simulink model "test_ab_to_ae"  (Simulink 7.6)
settings: Solver=ode45  StartTime=0.0  StopTime=500  RelTol=1e-3
libraries: simulink x18
settings Model: Creator=jporter  LastModifiedBy=jporter

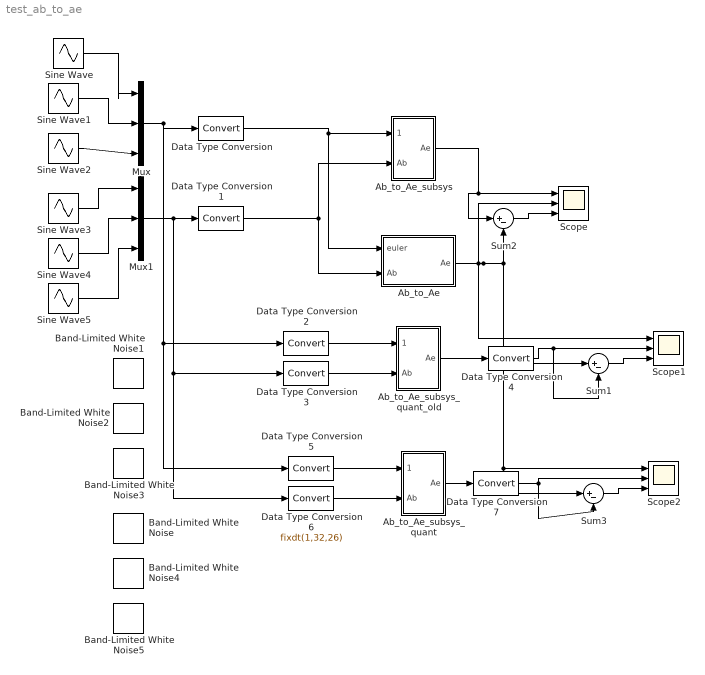
== system test_ab_to_ae ==
  Ab_to_Ae : Stateflow chart  TreatAsAtomicUnit=on
  Ab_to_Ae_subsys : Subsystem
  Ab_to_Ae_subsys_quant : Subsystem
  Ab_to_Ae_subsys_quant_old : Subsystem
  Band-Limited White Noise : simulink/Sources/Band-Limited White Noise  SystemSampleTime=-1  Cov=0.5  Ts=0.01  seed=[23341]
  Band-Limited White Noise{1..3,5} (4 alike) : simulink/Sources/Band-Limited White Noise  SystemSampleTime=-1  Cov=0  Ts=0.01  seed=[23341]
  Band-Limited White Noise4 : simulink/Sources/Band-Limited White Noise  SystemSampleTime=-1  Cov=0.5  Ts=0.01  seed=[23341]
  Data Type Conversion{,1..5,7} (7 alike) : DataTypeConversion
  Data Type Conversion6 : DataTypeConversion  OutDataTypeStr=fixdt(1,32,26)
  Mux : Mux  Inputs=3
  Mux1 : Mux  Inputs=3
  Scope : Scope  NumInputPorts=3
      settings: YMin=-5~-5~-5  YMax=5~5~5
  Scope1 : Scope  NumInputPorts=3
      settings: YMin=-1.5~-1.25~-2  YMax=1.5~0.75~1.5
  Scope2 : Scope  NumInputPorts=3
      settings: YMin=-1.25~-1.25~-7.5e-005  YMax=1.25~1.25~7.5e-005  SaveName=ScopeData2
  Sine Wave : Sin  SampleTime=0
  Sine Wave1 : Sin  Phase=1  SampleTime=0
  Sine Wave2 : Sin  Phase=2  SampleTime=0
  Sine Wave3 : Sin  Phase=3  SampleTime=0
  Sine Wave4 : Sin  Phase=4  SampleTime=0
  Sine Wave5 : Sin  Phase=5  SampleTime=0
  Sum1 : Sum  Inputs=|+-
  Sum2 : Sum  Inputs=|+-
  Sum3 : Sum  Inputs=|+-
  wires:
  Ab_to_Ae_subsys/1(Ae) -> Scope/1, Sum2/1
  Ab_to_Ae/1(Ae) -> Scope/2, Scope1/1, Sum2/2, Sum1/1, Scope2/1, Sum3/1
  Mux/1 -> Data Type Conversion/1, Data Type Conversion2/1, Data Type Conversion5/1
  Mux1/1 -> Data Type Conversion1/1, Data Type Conversion3/1, Data Type Conversion6/1
  Data Type Conversion/1 -> Ab_to_Ae_subsys/1(euler), Ab_to_Ae/1(euler)
  Data Type Conversion1/1 -> Ab_to_Ae/2(Ab), Ab_to_Ae_subsys/2(Ab)
  Sum2/1 -> Scope/3
  Sine Wave/1 -> Mux/1
  Sine Wave1/1 -> Mux/2
  Sine Wave2/1 -> Mux/3
  Sine Wave3/1 -> Mux1/1
  Sine Wave4/1 -> Mux1/2
  Sine Wave5/1 -> Mux1/3
  Data Type Conversion2/1 -> Ab_to_Ae_subsys_quant_old/1(euler)
  Data Type Conversion3/1 -> Ab_to_Ae_subsys_quant_old/2(Ab)
  Ab_to_Ae_subsys_quant_old/1(Ae) -> Data Type Conversion4/1
  Data Type Conversion4/1 -> Scope1/2, Sum1/2
  Sum1/1 -> Scope1/3
  Ab_to_Ae_subsys_quant/1(Ae) -> Data Type Conversion7/1
  Sum3/1 -> Scope2/3
  Data Type Conversion5/1 -> Ab_to_Ae_subsys_quant/1(euler1)
  Data Type Conversion6/1 -> Ab_to_Ae_subsys_quant/2(Ab)
  Data Type Conversion7/1 -> Scope2/2, Sum3/2

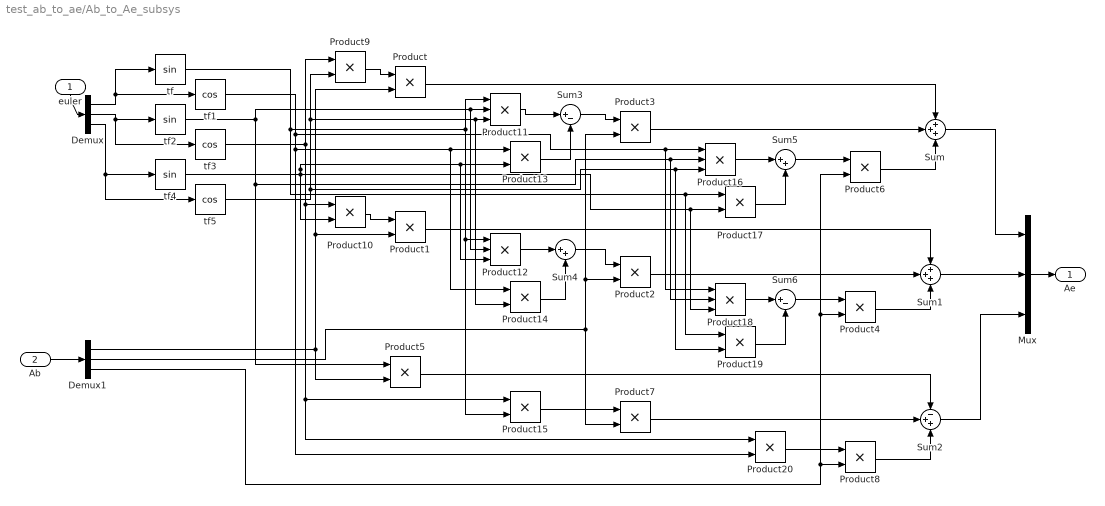
== system test_ab_to_ae/Ab_to_Ae_subsys ==
  euler : Inport
  Ab : Inport  Port=2
  Demux : Demux  Outputs=3
  Demux1 : Demux  Outputs=3
  Mux : Mux  Inputs=3
  Product{,1..10,13..15,17,19..20} (17 alike) : Product  RndMeth=Zero
  Product{11..12,16,18} (4 alike) : Product  Inputs=3  RndMeth=Zero
  Sum : Sum  Inputs=+++
  Sum1 : Sum  Inputs=+++
  Sum2 : Sum  Inputs=-++
  Sum3 : Sum  Inputs=|+-
  Sum4 : Sum  Inputs=|++
  Sum5 : Sum  Inputs=|++
  Sum6 : Sum  Inputs=|+-
  tf : Trigonometry
  tf1 : Trigonometry  Operator=cos
  tf2 : Trigonometry
  tf3 : Trigonometry  Operator=cos
  tf4 : Trigonometry
  tf5 : Trigonometry  Operator=cos
  Ae : Outport
  wires:
  Demux/1 -> tf/1, tf1/1
  Demux/2 -> tf2/1, tf3/1
  Demux/3 -> tf4/1, tf5/1
  Product/1 -> Sum/1
  Product3/1 -> Sum/2
  Product6/1 -> Sum/3
  Product1/1 -> Sum1/1
  Product2/1 -> Sum1/2
  Product4/1 -> Sum1/3
  Product5/1 -> Sum2/1
  Product7/1 -> Sum2/2
  Product8/1 -> Sum2/3
  tf3/1 -> Product9/1, Product10/1, Product15/1, Product20/1
  tf5/1 -> Product9/2, Product11/3, Product14/2, Product16/3, Product19/2
  Product9/1 -> Product/1
  Demux1/1 -> Product/2, Product1/2, Product5/2
  tf4/1 -> Product10/2, Product13/2, Product12/3, Product17/2, Product18/3
  Product10/1 -> Product1/1
  tf2/1 -> Product11/2, Product12/2, Product5/1, Product16/2, Product18/2
  Product11/1 -> Sum3/1
  tf/1 -> Product11/1, Product12/1, Product15/2, Product17/1, Product19/1
  tf1/1 -> Product16/1, Product18/1, Product13/1, Product14/1, Product20/2
  Product13/1 -> Sum3/2
  Sum3/1 -> Product3/1
  Demux1/2 -> Product3/2, Product2/2, Product7/2
  Product12/1 -> Sum4/1
  Product14/1 -> Sum4/2
  Sum4/1 -> Product2/1
  Product15/1 -> Product7/1
  Product16/1 -> Sum5/1
  Product17/1 -> Sum5/2
  Product18/1 -> Sum6/1
  Product19/1 -> Sum6/2
  Sum5/1 -> Product6/1
  Sum6/1 -> Product4/1
  Product20/1 -> Product8/1
  Demux1/3 -> Product8/2, Product4/2, Product6/2
  Sum/1 -> Mux/1
  Sum1/1 -> Mux/2
  Sum2/1 -> Mux/3
  euler/1 -> Demux/1
  Ab/1 -> Demux1/1
  Mux/1 -> Ae/1

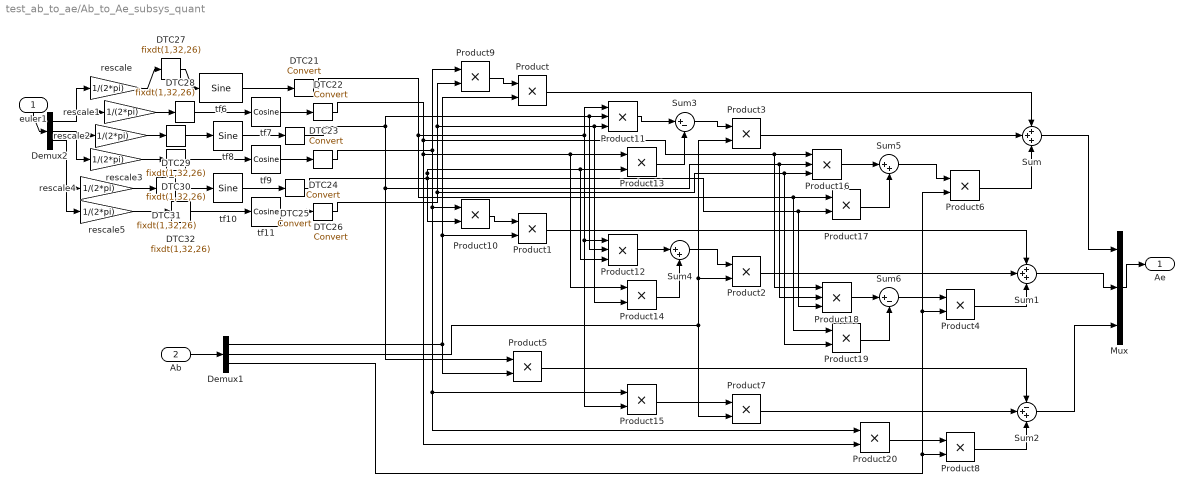
== system test_ab_to_ae/Ab_to_Ae_subsys_quant ==
  euler1 : Inport
  Ab : Inport  Port=2
  DTC{21..26} (6 alike) : DataTypeConversion
  DTC{27..32} (6 alike) : DataTypeConversion  OutDataTypeStr=fixdt(1,32,26)
  Demux1 : Demux  Outputs=3
  Demux2 : Demux  Outputs=3
  Mux : Mux  Inputs=3
  Product{,1..10,13..15,17,19..20} (17 alike) : Product  OutDataTypeStr=Inherit: Inherit via back propagation  RndMeth=Zero
  Product{11..12,16,18} (4 alike) : Product  Inputs=3  OutDataTypeStr=Inherit: Inherit via back propagation  RndMeth=Zero
  Sum : Sum  Inputs=+++  OutDataTypeStr=Inherit: Inherit via back propagation
  Sum1 : Sum  Inputs=+++  OutDataTypeStr=Inherit: Inherit via back propagation
  Sum2 : Sum  Inputs=-++  OutDataTypeStr=Inherit: Inherit via back propagation
  Sum3 : Sum  Inputs=|+-  OutDataTypeStr=Inherit: Inherit via back propagation
  Sum4 : Sum  Inputs=|++  OutDataTypeStr=Inherit: Inherit via back propagation
  Sum5 : Sum  Inputs=|++  OutDataTypeStr=Inherit: Inherit via back propagation
  Sum6 : Sum  Inputs=|+-  OutDataTypeStr=Inherit: Inherit via back propagation
  rescale{,1..5} (6 alike) : Gain  Gain=1/(2*pi)  ParamMin=1/(2*pi)  ParamMax=1/(2*pi)  OutDataTypeStr=fixdt(1,64,58)
  tf10 : simulink/Lookup Tables/Sine  SystemSampleTime=-1  Formula=sin(2*pi*u)  NumDataPoints=(2^7)+1  OutputWordLength=32
  tf11 : simulink/Lookup Tables/Cosine  SystemSampleTime=-1  Formula=cos(2*pi*u)  NumDataPoints=(2^7)+1  OutputWordLength=32
  tf6 : simulink/Lookup Tables/Sine  SystemSampleTime=-1  Formula=sin(2*pi*u)  NumDataPoints=(2^7)+1  OutputWordLength=32
  tf7 : simulink/Lookup Tables/Cosine  SystemSampleTime=-1  Formula=cos(2*pi*u)  NumDataPoints=(2^7)+1  OutputWordLength=32
  tf8 : simulink/Lookup Tables/Sine  SystemSampleTime=-1  Formula=sin(2*pi*u)  NumDataPoints=(2^7)+1  OutputWordLength=32
  tf9 : simulink/Lookup Tables/Cosine  SystemSampleTime=-1  Formula=cos(2*pi*u)  NumDataPoints=(2^7)+1  OutputWordLength=32
  Ae : Outport
  wires:
  Product/1 -> Sum/1
  Product3/1 -> Sum/2
  Product6/1 -> Sum/3
  Product1/1 -> Sum1/1
  Product2/1 -> Sum1/2
  Product4/1 -> Sum1/3
  Product5/1 -> Sum2/1
  Product7/1 -> Sum2/2
  Product8/1 -> Sum2/3
  DTC24/1 -> Product9/1, Product10/1, Product15/1, Product20/1
  DTC26/1 -> Product9/2, Product11/3, Product14/2, Product16/3, Product19/2
  Product9/1 -> Product/1
  Demux1/1 -> Product/2, Product1/2, Product5/2
  DTC25/1 -> Product10/2, Product13/2, Product12/3, Product17/2, Product18/3
  Product10/1 -> Product1/1
  DTC23/1 -> Product11/2, Product12/2, Product5/1, Product16/2, Product18/2
  Product11/1 -> Sum3/1
  DTC21/1 -> Product11/1, Product15/2, Product12/1, Product17/1, Product19/1
  DTC22/1 -> Product16/1, Product18/1, Product13/1, Product14/1, Product20/2
  Product13/1 -> Sum3/2
  Sum3/1 -> Product3/1
  Demux1/2 -> Product3/2, Product2/2, Product7/2
  Product12/1 -> Sum4/1
  Product14/1 -> Sum4/2
  Sum4/1 -> Product2/1
  Product15/1 -> Product7/1
  Product16/1 -> Sum5/1
  Product17/1 -> Sum5/2
  Product18/1 -> Sum6/1
  Product19/1 -> Sum6/2
  Sum5/1 -> Product6/1
  Sum6/1 -> Product4/1
  Product20/1 -> Product8/1
  Demux1/3 -> Product8/2, Product4/2, Product6/2
  Sum/1 -> Mux/1
  Sum1/1 -> Mux/2
  Sum2/1 -> Mux/3
  Ab/1 -> Demux1/1
  Mux/1 -> Ae/1
  Demux2/1 -> rescale/1, rescale1/1
  Demux2/2 -> rescale2/1, rescale3/1
  Demux2/3 -> rescale4/1, rescale5/1
  tf9/1 -> DTC24/1
  tf11/1 -> DTC26/1
  tf10/1 -> DTC25/1
  tf8/1 -> DTC23/1
  tf6/1 -> DTC21/1
  tf7/1 -> DTC22/1
  euler1/1 -> Demux2/1
  rescale/1 -> DTC27/1
  DTC27/1 -> tf6/1
  rescale1/1 -> DTC28/1
  DTC28/1 -> tf7/1
  rescale2/1 -> DTC29/1
  DTC29/1 -> tf8/1
  rescale3/1 -> DTC30/1
  DTC30/1 -> tf9/1
  rescale4/1 -> DTC31/1
  DTC31/1 -> tf10/1
  rescale5/1 -> DTC32/1
  DTC32/1 -> tf11/1

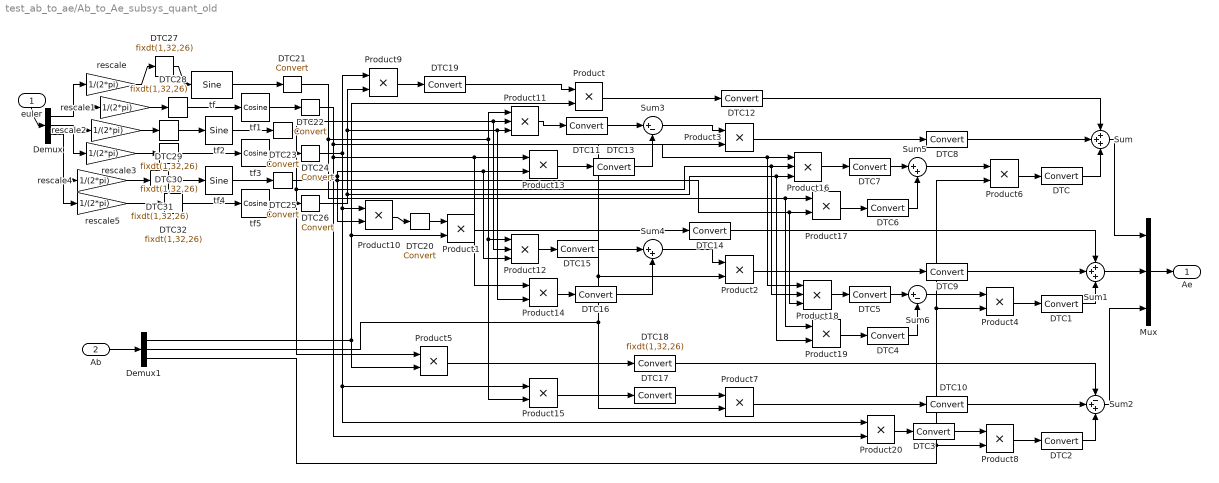
== system test_ab_to_ae/Ab_to_Ae_subsys_quant_old ==
  euler : Inport
  Ab : Inport  Port=2
  DTC{,1..17,19..26} (26 alike) : DataTypeConversion
  DTC{18,27..32} (7 alike) : DataTypeConversion  OutDataTypeStr=fixdt(1,32,26)
  Demux : Demux  Outputs=3
  Demux1 : Demux  Outputs=3
  Mux : Mux  Inputs=3
  Product : Product  OutDataTypeStr=fixdt(1,32,33)  RndMeth=Zero
  Product1 : Product  OutDataTypeStr=fixdt(1,32,34)  RndMeth=Zero
  Product{5,9..10,15} (4 alike) : Product  OutDataTypeStr=fixdt(1,64,52)  RndMeth=Zero
  Product11 : Product  Inputs=3  OutDataTypeStr=fixdt(1,64,52)  RndMeth=Zero
  Product12 : Product  Inputs=3  OutDataTypeStr=fixdt(1,32,41)  RndMeth=Zero
  Product13 : Product  OutDataTypeStr=fixdt(1,32,31)  RndMeth=Zero
  Product14 : Product  OutDataTypeStr=fixdt(1,32,30)  RndMeth=Zero
  Product16 : Product  Inputs=3  OutDataTypeStr=fixdt(1,32,35)  RndMeth=Zero
  Product17 : Product  OutDataTypeStr=fixdt(1,32,36)  RndMeth=Zero
  Product18 : Product  Inputs=3  OutDataTypeStr=fixdt(1,32,35)  RndMeth=Zero
  Product19 : Product  OutDataTypeStr=fixdt(1,32,35)  RndMeth=Zero
  Product2 : Product  OutDataTypeStr=fixdt(1,32,33)  RndMeth=Zero
  Product20 : Product  OutDataTypeStr=fixdt(1,32,30)  RndMeth=Zero
  Product3 : Product  OutDataTypeStr=fixdt(1,32,34)  RndMeth=Zero
  Product4 : Product  OutDataTypeStr=fixdt(1,32,39)  RndMeth=Zero
  Product6 : Product  OutDataTypeStr=fixdt(1,32,39)  RndMeth=Zero
  Product7 : Product  OutDataTypeStr=fixdt(1,32,38)  RndMeth=Zero
  Product8 : Product  OutDataTypeStr=fixdt(1,32,30)  RndMeth=Zero
  Sum : Sum  Inputs=+++  OutDataTypeStr=fixdt(1,32,30)
  Sum1 : Sum  Inputs=+++  OutDataTypeStr=fixdt(1,32,30)
  Sum2 : Sum  Inputs=-++  OutDataTypeStr=fixdt(1,32,30)
  Sum3 : Sum  Inputs=|+-  OutDataTypeStr=fixdt(1,32,31)
  Sum4 : Sum  Inputs=|++  OutDataTypeStr=fixdt(1,32,30)
  Sum5 : Sum  Inputs=|++  OutDataTypeStr=fixdt(1,32,36)
  Sum6 : Sum  Inputs=|+-  OutDataTypeStr=fixdt(1,32,35)
  rescale{,1..5} (6 alike) : Gain  Gain=1/(2*pi)  ParamMin=1/(2*pi)  ParamMax=1/(2*pi)  OutDataTypeStr=fixdt(1,64,58)
  tf : simulink/Lookup Tables/Sine  SystemSampleTime=-1  Formula=sin(2*pi*u)  NumDataPoints=(2^7)+1  OutputWordLength=32
  tf1 : simulink/Lookup Tables/Cosine  SystemSampleTime=-1  Formula=cos(2*pi*u)  NumDataPoints=(2^7)+1  OutputWordLength=32
  tf2 : simulink/Lookup Tables/Sine  SystemSampleTime=-1  Formula=sin(2*pi*u)  NumDataPoints=(2^7)+1  OutputWordLength=32
  tf3 : simulink/Lookup Tables/Cosine  SystemSampleTime=-1  Formula=cos(2*pi*u)  NumDataPoints=(2^7)+1  OutputWordLength=32
  tf4 : simulink/Lookup Tables/Sine  SystemSampleTime=-1  Formula=sin(2*pi*u)  NumDataPoints=(2^7)+1  OutputWordLength=32
  tf5 : simulink/Lookup Tables/Cosine  SystemSampleTime=-1  Formula=cos(2*pi*u)  NumDataPoints=(2^7)+1  OutputWordLength=32
  Ae : Outport
  wires:
  Demux/1 -> rescale/1, rescale1/1
  Demux/2 -> rescale2/1, rescale3/1
  Demux/3 -> rescale4/1, rescale5/1
  Product/1 -> DTC12/1
  Product3/1 -> DTC8/1
  Product6/1 -> DTC/1
  Product1/1 -> DTC14/1
  Product2/1 -> DTC9/1
  Product4/1 -> DTC1/1
  Product5/1 -> DTC18/1
  Product7/1 -> DTC10/1
  Product8/1 -> DTC2/1
  tf3/1 -> DTC24/1
  tf5/1 -> DTC26/1
  Product9/1 -> DTC19/1
  Demux1/1 -> Product/2, Product1/2, Product5/2
  tf4/1 -> DTC25/1
  Product10/1 -> DTC20/1
  tf2/1 -> DTC23/1
  Product11/1 -> DTC11/1
  tf/1 -> DTC21/1
  tf1/1 -> DTC22/1
  Product13/1 -> DTC13/1
  Sum3/1 -> Product3/1
  Demux1/2 -> Product3/2, Product2/2, Product7/2
  Product12/1 -> DTC15/1
  Product14/1 -> DTC16/1
  Sum4/1 -> Product2/1
  Product15/1 -> DTC17/1
  Product16/1 -> DTC7/1
  Product17/1 -> DTC6/1
  Product18/1 -> DTC5/1
  Product19/1 -> DTC4/1
  Sum5/1 -> Product6/1
  Sum6/1 -> Product4/1
  Product20/1 -> DTC3/1
  Demux1/3 -> Product8/2, Product4/2, Product6/2
  Sum/1 -> Mux/1
  Sum1/1 -> Mux/2
  Sum2/1 -> Mux/3
  euler/1 -> Demux/1
  Ab/1 -> Demux1/1
  Mux/1 -> Ae/1
  DTC/1 -> Sum/3
  DTC1/1 -> Sum1/3
  DTC2/1 -> Sum2/3
  DTC3/1 -> Product8/1
  DTC4/1 -> Sum6/2
  DTC5/1 -> Sum6/1
  DTC6/1 -> Sum5/2
  DTC7/1 -> Sum5/1
  DTC8/1 -> Sum/2
  DTC9/1 -> Sum1/2
  DTC10/1 -> Sum2/2
  DTC11/1 -> Sum3/1
  DTC12/1 -> Sum/1
  DTC13/1 -> Sum3/2
  DTC14/1 -> Sum1/1
  DTC15/1 -> Sum4/1
  DTC16/1 -> Sum4/2
  DTC17/1 -> Product7/1
  DTC18/1 -> Sum2/1
  DTC19/1 -> Product/1
  DTC20/1 -> Product1/1
  DTC21/1 -> Product11/1, Product15/2, Product12/1, Product17/1, Product19/1
  DTC22/1 -> Product16/1, Product18/1, Product13/1, Product14/1, Product20/2
  DTC23/1 -> Product11/2, Product12/2, Product5/1, Product16/2, Product18/2
  DTC24/1 -> Product9/1, Product10/1, Product15/1, Product20/1
  DTC25/1 -> Product10/2, Product13/2, Product12/3, Product17/2, Product18/3
  DTC26/1 -> Product9/2, Product11/3, Product14/2, Product16/3, Product19/2
  rescale/1 -> DTC27/1
  DTC27/1 -> tf/1
  rescale1/1 -> DTC28/1
  DTC28/1 -> tf1/1
  rescale2/1 -> DTC29/1
  DTC29/1 -> tf2/1
  rescale3/1 -> DTC30/1
  DTC30/1 -> tf3/1
  rescale4/1 -> DTC31/1
  DTC31/1 -> tf4/1
  rescale5/1 -> DTC32/1
  DTC32/1 -> tf5/1

== matlab function Ab_to_Ae ==
  data: euler input single size=[3]; Ae output single size=[3]; Ab input single size=[3]
function Ae = fcn(euler, Ab)
% This block supports the Embedded MATLAB subset.
% See the help menu for details. 
phi=euler(1);
theta=euler(2);
psi=euler(3);
c_phi=cos(phi);
c_theta=cos(theta);
c_psi=cos(psi);
s_phi=sin(phi);
s_theta=sin(theta);
s_psi=sin(psi);
R=single([c_theta*c_psi, c_theta*s_psi, -s_theta; s_phi*s_theta*c_psi-c_phi*s_psi, s_phi*s_theta*s_psi+c_phi*c_psi, c_theta*s_phi; c_phi*s_theta*c_psi+s_phi*s_psi, c_phi*s_theta*s_psi-s_phi*c_psi, c_theta*c_phi]);
%R=single(zeros(3,3));
%R(1,1)=c_theta*c_psi;
%R(1,2)=c_theta*s_psi;
%R(1,3)=-s_theta;
%R(2,1)=s_phi*s_theta*c_psi - c_phi*s_psi;
%R(2,2)=s_phi*s_theta*s_psi + c_phi*c_psi;
%R(2,3)=c_theta*s_phi;
%R(3,1)=c_phi*s_theta*c_psi + s_phi*s_psi;
%R(3,2)=c_phi*s_theta*s_psi - s_phi*c_psi;
%R(3,3)=c_theta*c_phi;
Ae= transpose(R) * Ab;
%Ae= single(Aed);
